simulink model "Validacion_angle"  (Simulink 8.8)
settings: Solver=VariableStepAuto  StartTime=0.0  StopTime=lim_sup  RelTol=1e-3
values from neighbouring files (symbols this model uses):
  k = -1.1735    [Validacion_datos_ROS.m]
  T = 0.05    [Validacion_datos_ROS.m]
  tau = 0.02833663927    [Validacion_datos_ROS.m]
undefined symbols (not defined in the file or in its folder): DiscIntNeverNeededParam
settings Model: Creator=Francisco José Mañas  LastModifiedBy=Francisco José Mañas
settings DataIOCC: LimitDataPoints=off  SaveFormat=Dataset  SignalLoggingSaveFormat=Dataset
settings OptimizationCC: LifeSpan=auto
settings DebuggingCC: UnderspecifiedInitializationDetection=Simplified  MergeDetectMultiDrivingBlocksExec=error  FcnCallInpInsideContextMsg=error  StateNameClashWarn=none  SFUnexpectedBacktrackingDiag=error  SFNoUnconditionalDefaultTransitionDiag=error  SFExecutionAtInitializationDiag=warning
settings HardwareCC: ProdBitPerPointer=64  ProdBitPerSizeT=64  ProdBitPerPtrDiffT=64  ProdLargestAtomicFloat=Float  ProdIntDivRoundTo=Zero  ProdEndianess=LittleEndian  ProdWordSize=64  ProdHWDeviceType=Intel->x86-64 (Windows64)
settings ModelReferenceCC: PropagateSignalLabelsOutOfModel=on
settings GRTTargetCC: TargetLangStandard=C99 (ISO)  GeneratePreprocessorConditionals=Use local settings  CombineOutputUpdateFcns=on  GRTInterface=off
settings ConfigComp: CovMetricSettings=dwe  CovHtmlReporting=off  CovSaveCumulativeToWorkspaceVar=off  CovSaveSingleToWorkspaceVar=off  CovExternalEMLEnable=on

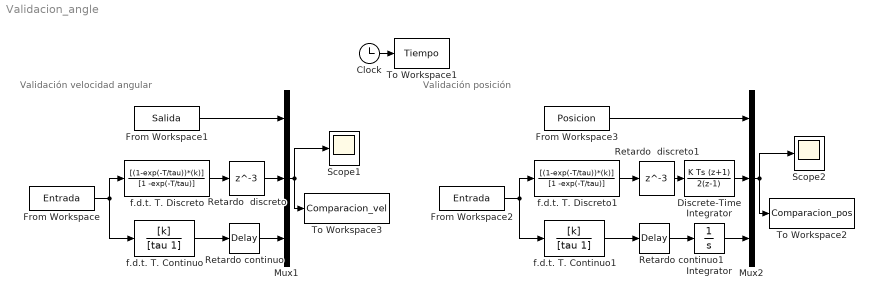
== system Validacion_angle ==
  note: Validación posición
  note: Validación velocidad angular
  Clock : Clock
  Discrete-Time Integrator : DiscreteIntegrator  IntegratorMethod=Integration: Trapezoidal  gainval=1  InitialConditionSetting=State (most efficient)  SampleTime=-1  ICPrevOutput=DiscIntNeverNeededParam  ICPrevScaledInput=DiscIntNeverNeededParam
  From Workspace : FromWorkspace  VariableName=Entrada  SampleTime=0
  From Workspace1 : FromWorkspace  VariableName=Salida  SampleTime=0
  From Workspace2 : FromWorkspace  VariableName=Entrada  SampleTime=0
  From Workspace3 : FromWorkspace  VariableName=Posicion  SampleTime=0
  Integrator : Integrator
  Mux1 : Mux  Inputs=3
  Mux2 : Mux  Inputs=3
  Retardo continuo : TransportDelay  DelayTime=0.15
  Retardo continuo1 : TransportDelay  DelayTime=0.15
  Retardo  discreto : Delay  DelayLength=3  SampleTime=T
  Retardo  discreto1 : Delay  DelayLength=3  SampleTime=T
  Scope1 : Scope
  Scope2 : Scope
  To Workspace1 : ToWorkspace  VariableName=Tiempo  SampleTime=-1
  To Workspace2 : ToWorkspace  VariableName=Comparacion_pos  SampleTime=-1
  To Workspace3 : ToWorkspace  VariableName=Comparacion_vel  SampleTime=-1
  f.d.t. T. Continuo : TransferFcn  Numerator=[k]  Denominator=[tau 1]
  f.d.t. T. Continuo1 : TransferFcn  Numerator=[k]  Denominator=[tau 1]
  f.d.t. T. Discreto : DiscreteTransferFcn  Numerator=[(1-exp(-T/tau))*(k)]  Denominator=[1 -exp(-T/tau)]  SampleTime=T
  f.d.t. T. Discreto1 : DiscreteTransferFcn  Numerator=[(1-exp(-T/tau))*(k)]  Denominator=[1 -exp(-T/tau)]  SampleTime=T
  wires:
  From Workspace1/1 -> Mux1/1
  From Workspace/1 -> f.d.t. T. Continuo/1, f.d.t. T. Discreto/1
  Clock/1 -> To Workspace1/1
  Retardo  discreto/1 -> Mux1/2
  Mux1/1 -> Scope1/1, To Workspace3/1
  f.d.t. T. Continuo/1 -> Retardo continuo/1
  Retardo continuo/1 -> Mux1/3
  f.d.t. T. Discreto/1 -> Retardo  discreto/1
  From Workspace3/1 -> Mux2/1
  From Workspace2/1 -> f.d.t. T. Continuo1/1, f.d.t. T. Discreto1/1
  Retardo  discreto1/1 -> Discrete-Time Integrator/1
  Mux2/1 -> Scope2/1, To Workspace2/1
  f.d.t. T. Continuo1/1 -> Retardo continuo1/1
  Retardo continuo1/1 -> Integrator/1
  f.d.t. T. Discreto1/1 -> Retardo  discreto1/1
  Integrator/1 -> Mux2/3
  Discrete-Time Integrator/1 -> Mux2/2
